simulink model "SinRange"  (R2022b)
settings: Solver=FixedStepDiscrete  StartTime=0.0  StopTime=10  FixedStep=0.001  RelTol=1e-3
libraries: simulink x1
settings Model: Creator=ZYH  LastModifiedBy=ZYH

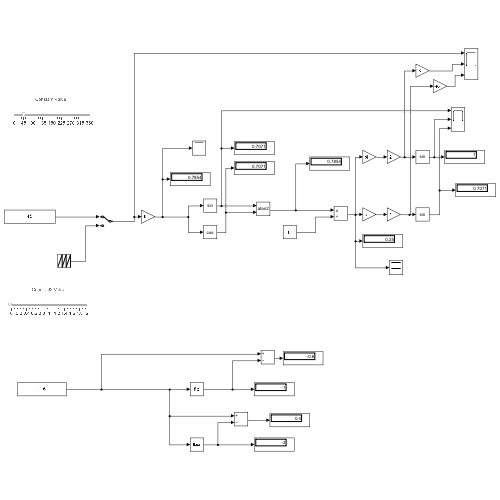
[thumbnail: Simulink's stored preview of the top-level diagram]
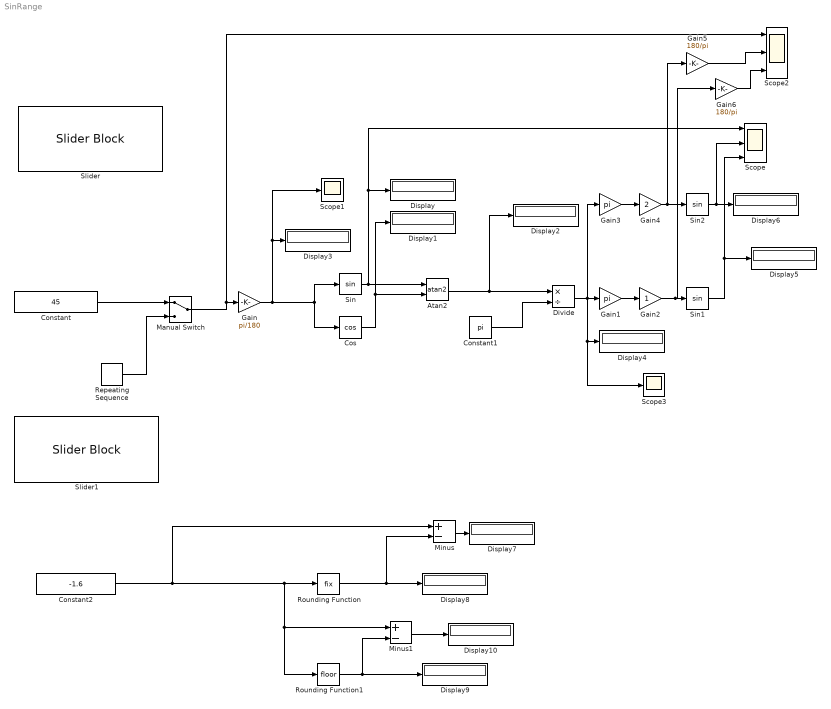
== system SinRange ==
  Atan2 : Trigonometry  Operator=atan2
  Constant : Constant  Value=45
  Constant1 : Constant  Value=pi
  Constant2 : Constant  Value=-1.6
  Cos : Trigonometry  Operator=cos
  Display{,1..10} (11 alike) : Display
  Divide : Product  Inputs=*/
  Gain : Gain  Gain=pi/180
  Gain1 : Gain  Gain=pi
  Gain2 : Gain
  Gain3 : Gain  Gain=pi
  Gain4 : Gain  Gain=2
  Gain5 : Gain  Gain=180/pi
  Gain6 : Gain  Gain=180/pi
  Manual Switch : ManualSwitch
  Minus : Sum  Inputs=+-
  Minus1 : Sum  Inputs=+-
  Repeating Sequence : simulink/Sources/Repeating Sequence  rep_seq_t=[0 2]  rep_seq_y=[0 360]
  Rounding Function : Rounding  Operator=fix
  Rounding Function1 : Rounding
  Scope : Scope  NumInputPorts=3
  Scope1 : Scope
  Scope2 : Scope  NumInputPorts=3
  Scope3 : Scope
  Sin : Trigonometry
  Sin1 : Trigonometry
  Sin2 : Trigonometry
  Slider : SliderBlock  ScaleMax=360
  Slider1 : SliderBlock  ScaleMax=2
  wires:
  Manual Switch/1 -> Scope2/1, Gain/1
  Gain/1 -> Display3/1, Scope1/1, Sin/1, Cos/1
  Cos/1 -> Atan2/2, Display1/1
  Sin/1 -> Atan2/1, Scope/1, Display/1
  Atan2/1 -> Display2/1, Divide/1
  Constant1/1 -> Divide/2
  Divide/1 -> Gain3/1, Gain1/1, Scope3/1, Display4/1
  Gain1/1 -> Gain2/1
  Sin1/1 -> Scope/3, Display5/1
  Gain2/1 -> Gain6/1, Sin1/1
  Sin2/1 -> Scope/2, Display6/1
  Gain3/1 -> Gain4/1
  Gain4/1 -> Gain5/1, Sin2/1
  Gain5/1 -> Scope2/2
  Gain6/1 -> Scope2/3
  Constant/1 -> Manual Switch/1
  Repeating Sequence/1 -> Manual Switch/2
  Constant2/1 -> Minus/1, Rounding Function1/1, Minus1/1, Rounding Function/1
  Rounding Function/1 -> Display8/1, Minus/2
  Minus/1 -> Display7/1
  Rounding Function1/1 -> Minus1/2, Display9/1
  Minus1/1 -> Display10/1
